simulink subsystem "power_windows_ECU_V6"  (R2021a)
settings: Solver=VariableStepAuto  StartTime=0.0  StopTime=10.0  RelTol=1e-3
settings Model: Creator=achu  LastModifiedBy=Sai229

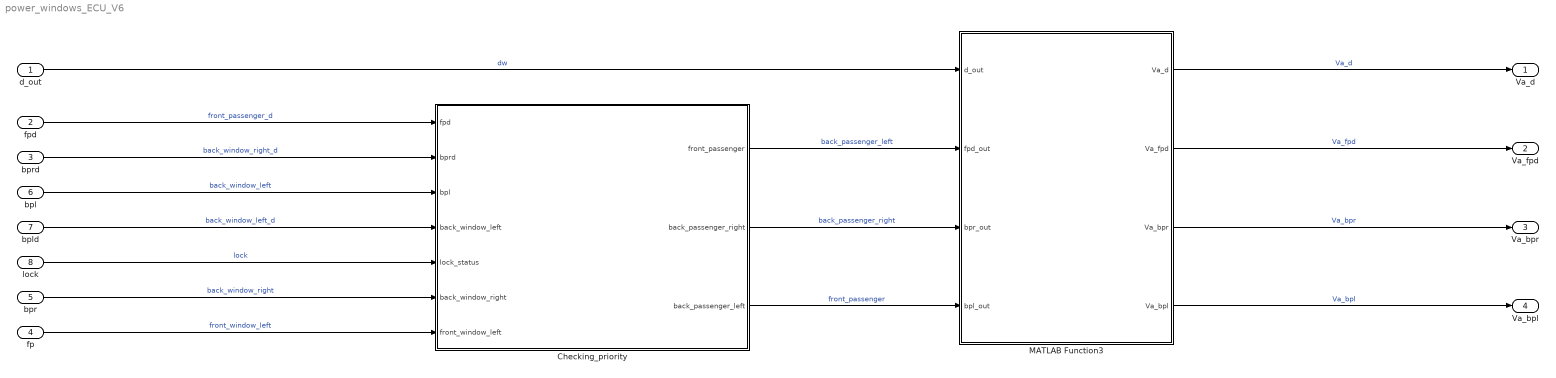
== system power_windows_ECU_V6 ==
  d_out : Inport
  fpd : Inport  Port=2
  bprd : Inport  Port=3
  fp : Inport  Port=4
  bpr : Inport  Port=5
  bpl : Inport  Port=6
  bpld : Inport  Port=7
  lock : Inport  Port=8
  Checking_priority : Subsystem  TreatAsAtomicUnit=on
      mask Display: disp("Priority check");
  MATLAB Function3 : MATLAB Function  TreatAsAtomicUnit=on
  Va_d : Outport
  Va_fpd : Outport  Port=2
  Va_bpr : Outport  Port=3
  Va_bpl : Outport  Port=4
  wires:
  MATLAB Function3/4(Va_bpl) -> Va_bpl/1  "Va_bpl"
  bpl/1 -> Checking_priority/3(bpl)  "back_window_left"
  bprd/1 -> Checking_priority/2(bprd)  "back_window_right_d"
  MATLAB Function3/1(Va_d) -> Va_d/1  "Va_d"
  MATLAB Function3/3(Va_bpr) -> Va_bpr/1  "Va_bpr"
  bpld/1 -> Checking_priority/4(back_window_left)  "back_window_left_d"
  bpr/1 -> Checking_priority/6(back_window_right)  "back_window_right"
  MATLAB Function3/2(Va_fpd) -> Va_fpd/1  "Va_fpd"
  lock/1 -> Checking_priority/5(lock_status)  "lock"
  fpd/1 -> Checking_priority/1(fpd)  "front_passenger_d"
  d_out/1 -> MATLAB Function3/1(d_out)  "dw"
  fp/1 -> Checking_priority/7(front_window_left)  "front_window_left"
  Checking_priority/1(front_passenger) -> MATLAB Function3/2(fpd_out)  "back_passenger_left"
  Checking_priority/2(back_passenger_right) -> MATLAB Function3/3(bpr_out)  "back_passenger_right"
  Checking_priority/3(back_passenger_left) -> MATLAB Function3/4(bpl_out)  "front_passenger"

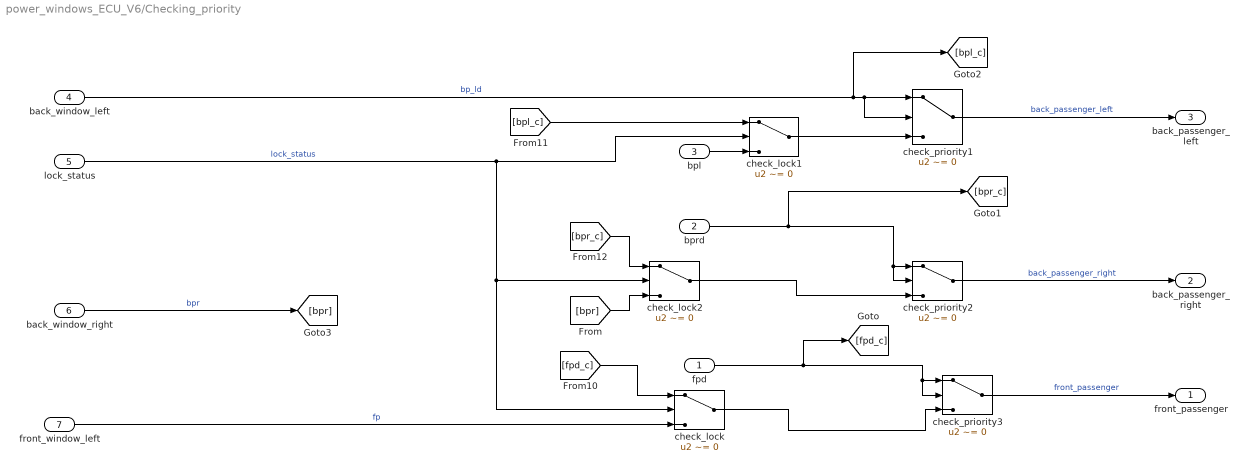
== system power_windows_ECU_V6/Checking_priority ==
  fpd : Inport
  bprd : Inport  Port=2
  bpl : Inport  Port=3
  back_window_left : Inport  Port=4
  lock_status : Inport  Port=5
  back_window_right : Inport  Port=6
  front_window_left : Inport  Port=7
  check_lock : Switch  Criteria=u2 ~= 0
  check_lock1 : Switch  Criteria=u2 ~= 0
  check_lock2 : Switch  Criteria=u2 ~= 0
  check_priority1 : Switch  Criteria=u2 ~= 0
  check_priority2 : Switch  Criteria=u2 ~= 0
  check_priority3 : Switch  Criteria=u2 ~= 0
  front_passenger : Outport
  back_passenger_right : Outport  Port=2
  back_passenger_left : Outport  Port=3
  wires:
  front_window_left/1 -> check_lock/3  "fp"
  back_window_right/1 -> [bpr]  "bpr"
  lock_status/1 -> check_lock1/2, check_lock2/2, check_lock/2  "lock_status"
  check_priority3/1 -> front_passenger/1  "front_passenger"
  check_priority2/1 -> back_passenger_right/1  "back_passenger_right"
  check_priority1/1 -> back_passenger_left/1  "back_passenger_left"
  back_window_left/1 -> check_priority1/2, check_priority1/1, [bpl_c]  "bp_ld"
  [bpr] -> check_lock2/3
  fpd/1 -> [fpd_c], check_priority3/2, check_priority3/1
  bprd/1 -> [bpr_c], check_priority2/2, check_priority2/1
  [fpd_c] -> check_lock/1
  check_lock1/1 -> check_priority1/3
  [bpl_c] -> check_lock1/1
  check_lock2/1 -> check_priority2/3
  bpl/1 -> check_lock1/3
  [bpr_c] -> check_lock2/1
  check_lock/1 -> check_priority3/3

== matlab function power_windows_ECU_V6/MATLAB Function3 ==
  data: d_out input; Va_d output; fpd_out input; bpr_out input; bpl_out input; Va_fpd output; Va_bpr output; Va_bpl output
function [Va_d,Va_fpd, Va_bpr, Va_bpl] = fcn(d_out, fpd_out, bpr_out, bpl_out)
dout=0;
fpd=0;
bpr=0;
bpl=0;
if (d_out==1)
    dout=20;
elseif (d_out==-1)
    dout=-20;
elseif (d_out==0)
    dout=0;
end

if (fpd_out==1)
        fpd=20;
elseif (fpd_out==-1)
    fpd=-20;
elseif (fpd_out==0)
    fpd=0;
end

if (bpr_out==1)
        bpr=20;
elseif (bpr_out==-1)
    bpr=-20;
elseif (bpr_out==0)
    bpr=0;
end

if (bpl_out==1)
        bpl=20;
elseif (bpl_out==-1)
    bpl=-20;
elseif (bpl_out==0)
    bpl=0;
end
  
Va_d = dout;
Va_fpd = fpd;
Va_bpr=bpr;
Va_bpl=bpl;
